simulink subsystem "PvtSubSys_HMI"  (R2020b)
settings: Solver=VariableStepAuto  StartTime=0.0  StopTime=10.0  RelTol=1e-3
undefined symbols (not defined in the file): P_HMI_LDW_LKAWarnTime, P_HMI_ObjectTypeFilter, P_HMI_WarnFormLDWReq
libraries: simulink x212, TrueDurationTime x6
(part 3 of 8)

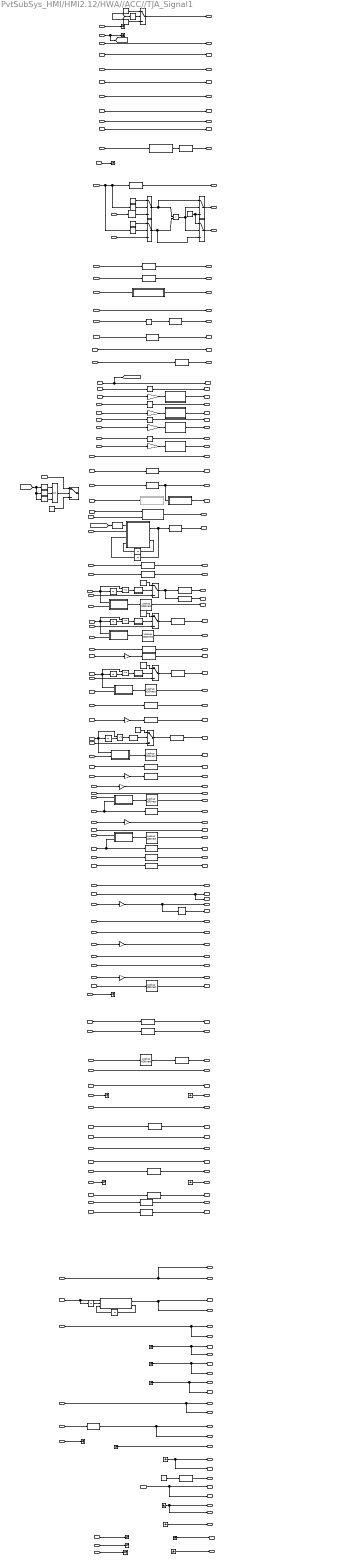
== system PvtSubSys_HMI/HMI2.12/HWA//ACC//TJA_Signal1 ==
  note: P O3目标是否存在
  note: 0x0:OFF
      | 0x1:ON
  note: 0x0:No Request
      | 0x1:Request
  note: 0x0:No Request
      | 0x1:Request
  note: 是否存在ACC 主目标PO0
  note: P O0目标是否存在
      | 仪表用ACC_RlvTgtDetn信号作为判断 目标是否存在
  note: 0=Obj_Type_INVALIDE |
      | 1=Obj_Type_UnknownType |
      | 2=Obj_Type_CAR |
      | 3=Obj_Type_TRUCK |
      | 4=Obj_Type_MOTORBIKE |
      | 5=Obj_Type_BICYCLE |
      | 6=Obj_Type_PEDESTRIAN |
      | 7=Obj_Type_GENERAL_OBJECT |
      | 8=Obj_Type_ANIMAL|
  note: DEFAULT(7)
  note: 0x0:No TakeOver request
      | 0x1:Valid TakeOver request
  note: 0x0:Fuction Not  Available
      | 0x1:Fuction Available
      | 0x2:Performance degradation(融合)
      | 0x3:Reserved
  note: 0x0:No display
      | 0x1:Distance_1 one bar
      | 0x2:Distance_2 two bars
      | 0x3:Distance_3 three bars
      | 0x4:Distance_4 four bars
      | 0x5-0x7:Resvered
  note: 0x0:No Display
      | 0x1:Override
      | 0x2:Deceleration
      | 0x3:Reserved
  note: 0x00:No display
      | 0x01:Unable to activate ACC due to speed not achive
      | 0x02:ACC active control is cancelled
      | 0x03:Resvered
      | 0x04:ACC and PEBS temporary unavailable
      | 0x05:Unable to activate ACC due to other limitation(except speed not achive)
      | 0x06:ACC and PEBS error
      | 0x07:ACC temporary unavailable
      | 0x08:Resvered
      | 0x09:Blindness
      | 0x0A-0x1F:Resvered
  note: 0x0:No display
      | 0x1:Unable to activate TJA/ICA due to other limitation
      | 0x2:TJA/ICA active control is cancelled
      | 0x3:TJA/ICA   temporarily unavailable
      | 0x4:Current IGN Cycle Function Inhibit
      | 0x5-0x7:Resvered
  note: 0x0:OFF mode
      | 0x1:Idle mode
      | 0x2:Ready mode
      | 0x3:Active
      | 0x4:Reserved
      | 0x5:Warning Level 1
      | 0x6:Warning Level 2
      | 0x7:Warning Level 3
      | 0x8:Reserved
      | 0x9:Failure
      | 0xA-0xF:Reserved
  note: 0x0:No display
      | 0x1:Unable to activate CruiseChauffer due to other limitation
      | 0x2:CruiseChauffer active control is cancelled
      | 0x3:CruiseChauffer temporarily unavailable
      | 0x4:Take over request
      | 0x5:Current IGN Cycle Function Inhibit
      | 0x6: Please Keep Attention
      | 0x7:To cross the tunnel, please take over  in time
      | 0x8:Have a branch road ahead. Please take over in time
      | 0x9-0xF:Reserved
  note: 0x0:No display
      | 0x1:TimeGap_1 1s
      | 0x2:TimeGap_2 1.4s
      | 0x3:TimeGap_3 1.8s
      | 0x4:TimeGap_4 2.1s
      | 0x5-0x7:Reserved
  note: 0x0:No object
      | 0x1:Target object detected
  note: 0x0:Not dectected
      | 0x1:Dectected
      | 0x2:Reserved
      | 0x3:Invalid
  note: 0x0:OFF mode
      | 0x1:Passive mode
      | 0x2:Active mode
      | 0x3:Reserved
      | 0x4: Failure
      | 0x5-0x7: Reserved
  note: 3 off
      | 0 off_selected
      | 1 acc_selected
      | 2 tja_seclected
      | 4 acc_on
      | 5 tja_on
  note: 0x0:No Warning
      | 0x1:Warning Level 1
      | 0x2:Warning Level 2
      | 0x3:Warning Level 3
  note: 0x0:No display
      | 0x1:Unable to activate HWA due to other limitation
      | 0x2:HWA active control is cancelled
      | 0x3:Turn off the turn light
      | 0x4:Active confirm
      | 0x5:Overtime for lane change
      | 0x6:lane change is cancelled
      | 0x7:HWA temporary unavailable
      | 0x8:Speed is too low to support lane change
      | 0x9:HWA need to restart the engine
      | 0xA:Take over request
      | 0xB: Please Keep Attention
      | 0xC:To cross the tunnel, please take over  in time
      | 0xD:Have a branch road ahead. Please take over in time
      | 0xE-0xF:Reserve
  note: FD2
      | 0x0:No display
      | 0x1:left satisfied
      | 0x2:right satisfied
      | 0x3:left not satisfied
      | 0x4:right not satisfied
      | 0x5~0x7:reserved
  note: FD2
      | 0x0:No display
      | 0x1:left
      | 0x2:right
      | 0x3:reserved
  note: 0x0:OFF mode
      | 0x1:Passive mode(Reject)
      | 0x2:Passive mode(Stand-by)
      | 0x3:Active-Control mode
      | 0x4:Brake-only mode
      | 0x5:Override
      | 0X6:Standstill
      | 0x7:Failure mode Longctrl
      | 0x8:Reserved
      | 0x9:Shut off
      | 0xA~0xF:Reserved
  note: 0x0:No Request
      | 0x1:Request
  note: ACC起步请求标志位
  note: 0x0:No request
      | 0x1:Request park Shift
      | 0x2:Invalid
      | 0x3:Reserved
  note: 1：park
      | 0：no
  note: 0x0:Not active
      | 0x1:AEB active
      | 0x2:Safestop active
      | 0x3:Reserved
  note: 0x0: No Display
      | 0x1: HOD Level 1
      | 0x2: HOD Level 2
      | 0x3: DAM Warning
      | 0x4-0x7:Resvered
  note: Diver Hands-on detection warning and
      | Driver Attention warning
  note: 0x0:Normal
      | 0x1:High sensitivity
      | 0x2:Low sensitivity
      | 0x3:Reserved
  note: 需要修改coding
  note: 状态机
  note: 0：preceding
      | 1： oncoming
  note: 前方300m（暂定）弯道曲率
  note: 0x0 00-0x1FE:Valid Value(Left bend)
      | 0x1 FF:Straightaway
      | 0x2 00-0x3FD:Valid Value((Reft bend))
      | 0x3 FE:Reserved
      | 0x3 FF:Unknown
  note: Current position curvature
  note: 当前位置道路曲率
  note: Object_Type
  note: ACC主目标：ACCTarget objective and Video Camera Fusion
      | 0x0:No Fusion
      | 0x1:Fusion
  note: 0x0:Not active
      | 0x1:Active
  note: coding值oncoming规划到Reseved
  note: 0x0:No display
      | 0x1:Automatic lane change function failure
      | 0x2-0x3:Reserve
  note: 黄色：ACC_FD2
      | 绿色：ACC_FD1
  note: 0x0=Frader前雷达
      | 0x1=Fcamera前摄像头
      | 0x2=LFRadar左前雷达
      | 0x3=RFRadar右前雷达
      | 0x4=RLRader左后雷达
      | 0x5=RRRader 右后
      | 0x6=FRadCamFusion前雷达和摄像头
      | 0x7=FRadCamLRadFusion前雷达摄像头左前
      | 0x8=FRadCamRRadFusion前雷达摄像头右前
      | 0x9=FRadCamRRadLRadFusion前雷达摄像头左前右前
      | 0x10=FRadLRadFusion 前雷达左前
      | 0x11=FRadRRadFusion前雷达右前
      | 0x12=FRadLRadRRadFusion前雷达右前左前
      | 0x13=LRadRRadFusion 右前左前
      | 0x14=OtherFusion
  note: 0x0:Unknown
      | 0x1:Emergency lane
      | 0x2:Single-lane road
      | 0x3:Left-most lane
      | 0x4:Right-most lane
      | 0x5:One of middle lanes on road with three or more lanes
      | 0x6:Reserved
      | 0x7:Invalid data
  note: Lateral distance of the second target in left lane
  note: 0x0:Unkown
      | 0x1:Sedan
      | 0x2:Truck
      | 0x3:Motorcycle
      | 0x4:Pedestrian
      | 0x5:Bicycle
      | 0x6:Reserved
      | 0x7:Invalid
  note: 0x0:Not dectected
      | 0x1:Dectected
      | 0x2:Reserved
      | 0x3:Invalid
  note: 0x0:No Request
      | 0x1:Request
  note: 0x0:No Response
      | 0X1:Response
  note: 核实后：雷达 故障的时候发invalid
  note: SpdLim_Long_Distance
  note: 0x0:OFF
      | 0X1:ON
  note: 0x0:UNDEFINED
      | 0x1:PRECEDING
      | 0x2:STATIONARY
      | 0x3:STOPPED
      | 0x4-0x7:Reserved
  note: 0x0:Unkown
      | 0x1:Sedan
      | 0x2:Truck
      | 0x3:Motorcycle
      | 0x4:Pedestrian
      | 0x5:Bicycle
      | 0x6:Reserved
      | 0x7:Invalid
  note: error=invalid
  note: 0x0:No display
      | 0x1:Distance_1 one bar
      | 0x2:Distance_2 two bars
      | 0x3:Distance_3 three bars
      | 0x4:Distance_4 four bars
      | 0x5-0x7:Resvered
  note: 0x0:off
      | 0x1:ACC selected
      | 0x2:TJA/ICA selected
      | 0x3:Off selected
      | 0x4:ACC on
      | 0x5:TJA/ICA on
      | 0x6-0x7:Reserved
  note: 0x0:no fusion
      | 0x1:fusion
  note: 0x0:OFF
      | 0x1:ON
  note: 0x0:off
      | 0x1:ACC selected
      | 0x2:TJA/ICA selected
      | 0x3:Off selected
      | 0x4:ACC on
      | 0x5:TJA/ICA on
      | 0x6-0x7:Reserved
  note: 0x0:inactive0x1:active
  note: 0x0:Unkown
      | 0x1:Sedan
      | 0x2:Truck
      | 0x3:Motorcycle
      | 0x4:Pedestrian
      | 0x5:Bicycle
      | 0x6:Reserved
      | 0x7:Invalid
  note: 0x0:No display
      | 0x1:Speed Limit Confirm Request
      | 0x2:Speed Limit Take Over Request
      | 0x3:Reduce speed on a curve(过弯安全降速)
  note: 0=Obj_MovType_INVALID |
      | 1=Obj_MovType_UNKNOWN |
      | 2=Obj_MovType_MOVING |
      | 3=Obj_MovType_STATIONARY |
      | 4=Obj_MovType_STOPPED|
      | 5= Obj_MovType_MOVING_SLOWLY
  note: 0x0:Unknown
      | 0x1:Hands off
      | 0x2:Not hands off
      | 0x3:Reserved
  note: 0x0:no request
      | 0x1:The front car has started
      | 0x2:The front car has started,Please pay attention to the road environmentahead
      | 0x3:The front car has started,please keep your attention
      | 0x4:The front car has started,please take over the car
      | 0x5-0x7:Reserved
  note: 0x0:Good
      | 0x1:Unbelievable
      | 0x2:Low
      | 0x3:Middle
      | 0x4:High Level 1
      | 0x5:High Level 2
  note: 0x0:No warning
      | 0x1:Level1 warning
      | 0x2:Level2 warning
      | 0x3:Level3 warning
      | 0x4:Level4 warning
      | 0x5:Level5 warning
      | 0x6-0x7:Reserved
  note: HWAWarnig优先级最高，可屏蔽其他两者；Handsoffwarn和DrvrSts谁高报谁，一样则报Handsoff；
  note: 0x0:Turn OFF
      | 0x1:Turn Left ON
      | 0x2:Turn Right ON
  ACCSts : Inport
  TJASts : Inport  Port=2
  HWASts : Inport  Port=3
  ACC_ModeDisp : Inport  Port=4
  TJA_ModeDisp : Inport  Port=5
  HWA_ModeDisp : Inport  Port=6
  ACCTextDisp : Inport  Port=7
  TJATextDisp : Inport  Port=8
  ALC_Resp : Inport  Port=9
  HWA_Resp : Inport  Port=10
  HWAWarningLevel : Inport  Port=11
  ACC_TimeGapSet : Inport  Port=12
  ACC_SpdSetValue : Inport  Port=13
  TJA_ACC_SelSts : Inport  Port=14
  ACC_TakeOverReq : Inport  Port=15
  ACC_HazActv : Inport  Port=16
  IntelligentCurveActive : Inport  Port=17
  fu_typeP0 : Inport  Port=18
  P0HeadingAngle : Inport  Port=19
  fu_typeP2 : Inport  Port=20
  P2HeadingAngle : Inport  Port=21
  fu_typeP3 : Inport  Port=22
  P3HeadingAngle : Inport  Port=23
  fu_typeP1 : Inport  Port=24
  P1HeadingAngle : Inport  Port=25
  DriverInloop_Monitor : Inport  Port=26
  HWA_SnvtySet_Resp : Inport  Port=27
  HWA_LaneChangeReq : Inport  Port=28
  ACC_Decel_Req : Inport  Port=29
  ACC_ISLResp : Inport  Port=30
  ICA_HandsOffSwtResp : Inport  Port=31
  targetExistP0 : Inport  Port=32
  ObjTypeP0 : Inport  Port=33
  targetExistP1 : Inport  Port=34
  ObjTypeP1 : Inport  Port=35
  dxP1 : Inport  Port=36
  ObjDYP1 : Inport  Port=37
  targetExistP2 : Inport  Port=38
  ObjTypeP2 : Inport  Port=39
  dxP2 : Inport  Port=40
  ObjDYP2 : Inport  Port=41
  targetExistP3 : Inport  Port=42
  ObjTypeP3 : Inport  Port=43
  dxP3 : Inport  Port=44
  ObjDYP3 : Inport  Port=45
  ISL_InterSysInfoDisp : Inport  Port=46
  ACC_DrvOffReq : Inport  Port=47
  IDP2 : Inport  Port=48
  IDP1 : Inport  Port=49
  IDP3 : Inport  Port=50
  ACC_Decel_ReqValue : Inport  Port=51
  ACC_ParkShiftReq : Inport  Port=52
  HCUTrqReqActive : Inport  Port=53
  CCTextDisp : Inport  Port=54
  dyP4 : Inport  Port=55
  dxP4 : Inport  Port=56
  ObjTypeP4 : Inport  Port=57
  targetExistP4 : Inport  Port=58
  dyP5 : Inport  Port=59
  dxP5 : Inport  Port=60
  ObjTypeP5 : Inport  Port=61
  targetExistP5 : Inport  Port=62
  IDP0 : Inport  Port=63
  dxP0 : Inport  Port=64
  ObjDYP0 : Inport  Port=65
  ACCTgtObjObstcl : Inport  Port=66
  ACCTgtObjExist : Inport  Port=67
  ACCTgtObjVy : Inport  Port=68
  vxRelP0 : Inport  Port=69
  axAbsGroundP0 : Inport  Port=70
  ACCTgtObjAy : Inport  Port=71
  ObjMovingStateP0 : Inport  Port=72
  Object_Orientation : Inport  Port=73
  ACCTgtObjCntAlive : Inport  Port=74
  HandsoffDetd : Inport  Port=75
  DrivingOnHighWay : Inport  Port=76
  dRoadCurvature : Inport  Port=77
  TSR_Sign_Long_Distance : Inport  Port=78
  RoadCurvatureFar : Inport  Port=79
  RampDistance : Inport  Port=80
  NavSpdLimValue : Inport  Port=81
  RoadCurvatureFarDistance : Inport  Port=82
  NavSpdLimUnit_HUT : Inport  Port=83
  TunnelDistance : Inport  Port=84
  ADAS_Posn_CurLane : Inport  Port=85
  BridgeDistance : Inport  Port=86
  ACC_SOS_Req : Inport  Port=87
  MapDataValid : Inport  Port=88
  DrvrState : Inport  Port=89
  "Inter_AEB_TgtDecel_Req " : Inport  Port=90
  Inter_FCW_Warn : Inport  Port=91
  CruiseChauffeur_ModeDisp : Inport  Port=92
  HWATextDisp : Inport  Port=93
  HandsOffWarningLevel : Inport  Port=94
  ACC_TgtObjBarDisp1 : Inport  Port=95
  ACC_LeTgtObjBarDisp1 : Inport  Port=96
  ACC_RiTgtObjBarDisp1 : Inport  Port=97
  HWA_TurnLightReq : Inport  Port=98
  ACC_DrvrOffDisp : Inport  Port=99
  100ms1 : Subsystem
  100ms2 : Subsystem
  100ms3 : Subsystem
  100ms4 : Subsystem
  ACCSts1 : InportShadow
  ACCSts2 : InportShadow
  ACCSts4 : InportShadow
  ACC_Decel_Req1 : InportShadow  Port=29
  Compare To Constant : simulink/Logic and Bit Operations/Compare To Constant  relop=~=  const=7  OutDataTypeStr=boolean
  Compare To Constant{1..6} (6 alike) : simulink/Logic and Bit Operations/Compare To Constant  relop=~=  const=0  OutDataTypeStr=boolean
  Compare To Constant10 : simulink/Logic and Bit Operations/Compare To Constant  relop===  const=7  OutDataTypeStr=boolean
  Compare To Constant7 : simulink/Logic and Bit Operations/Compare To Constant  relop===  const=3  OutDataTypeStr=boolean
  Compare To Constant8 : simulink/Logic and Bit Operations/Compare To Constant  relop===  const=5  OutDataTypeStr=boolean
  Compare To Constant9 : simulink/Logic and Bit Operations/Compare To Constant  relop===  const=6  OutDataTypeStr=boolean
  Constant{,1..2,10} (4 alike) : Constant  Value=0  OutDataTypeStr=uint8
  Constant3 : Constant
  Constant4 : Constant  Value=0
  Constant{5..8} (4 alike) : Constant  Value=0  OutDataTypeStr=boolean
  Constant9 : Constant  OutDataTypeStr=uint8
  Data Type Conversion{,1..30,34,36} (33 alike) : DataTypeConversion
  Data Type Conversion31 : DataTypeConversion  OutDataTypeStr=uint16
  Data Type Conversion32 : DataTypeConversion  OutDataTypeStr=uint16
  Data Type Conversion33 : DataTypeConversion  OutDataTypeStr=uint16
  Data Type Conversion35 : DataTypeConversion  OutDataTypeStr=uint8
  Detect Increase23 : simulink/Logic and Bit Operations/Detect Increase  vinit=0.0  OutDataTypeStr=boolean
  Direct Lookup Table (n-D){,1..3,8..9} (6 alike) : LookupNDDirect  NumberOfTableDimensions=1  Table=[7 0 1 2 3 5 4 0 0]  TableDataTypeStr=uint8
  Direct Lookup Table (n-D)10 : LookupNDDirect  NumberOfTableDimensions=1  Table=[1 0 1 2 3 4 1 2 3 4]  TableDataTypeStr=uint8
  Direct Lookup Table (n-D)4 : LookupNDDirect  NumberOfTableDimensions=1  Table=[0 0 1 2 3 1]  TableDataTypeStr=uint8
  Direct Lookup Table (n-D)5 : LookupNDDirect  NumberOfTableDimensions=1  Table=[2 1]  TableDataTypeStr=uint8
  Enlong3s : Subsystem
  Gain{,1..3} (4 alike) : Gain  Gain=-1/57.3  OutDataTypeStr=Inherit: Same as input
  Gain{4..11} (8 alike) : Gain  Gain=-1  OutDataTypeStr=Inherit: Same as input
  Ground{,1,3..8,12,14,20} (11 alike) : Ground
  HWASts1 : InportShadow  Port=3
  IDP0copy : InportShadow  Port=63
  Logical Operator : Logic  Operator=OR  Inputs=3  AllPortsSameDT=off  OutDataTypeStr=boolean
  MATLAB Function : MATLAB Function  TreatAsAtomicUnit=on
  MATLAB Function1 : MATLAB Function  TreatAsAtomicUnit=on
  MATLAB Function2 : MATLAB Function  TreatAsAtomicUnit=on
  MATLAB Function3 : MATLAB Function  Commented=on  TreatAsAtomicUnit=on
  MATLAB Function4 : MATLAB Function  TreatAsAtomicUnit=on
  MATLAB Function5 : MATLAB Function  TreatAsAtomicUnit=on
  MATLAB Function6 : MATLAB Function  TreatAsAtomicUnit=on
  MATLAB Function7 : MATLAB Function  TreatAsAtomicUnit=on
  MATLAB Function8 : MATLAB Function  TreatAsAtomicUnit=on
  MATLAB Function9 : MATLAB Function  TreatAsAtomicUnit=on
  Relational Operator : RelationalOperator  Operator=>  OutDataTypeStr=boolean  RndMeth=Simplest
  Relational Operator{1..4} (4 alike) : RelationalOperator  Operator=~=  OutDataTypeStr=boolean  RndMeth=Simplest
  Signal Copy : SignalConversion  OverrideOpt=off
  Subsystem : Subsystem
  Subsystem1 : Subsystem
  Subsystem2 : Subsystem
  Subsystem3 : Subsystem
  Subsystem4 : Subsystem
  Subsystem5 : Subsystem
  Switch{,1..8} (9 alike) : Switch  Criteria=u2 ~= 0
  Switch9 : Switch  Criteria=u2 > Threshold
  Terminator{,1..6,16,18,22} (10 alike) : Terminator
  Unit Delay{,1..7} (8 alike) : UnitDelay  SampleTime=-1  HasFrameUpgradeWarning=on
  fu_typeP4 : InportShadow  Port=18
  vxRelP01 : InportShadow  Port=69
  ALC_InterSysInfoDisp : Outport
  ACC_ModDisp : Outport  Port=2
  TJA_ICA_ModDisp : Outport  Port=3
  HWA_InterSysInfoDisp : Outport  Port=4
  HWA_ModDisp : Outport  Port=5
  ACC_InterSysInfoDisp : Outport  Port=6
  TJA_ICA_InterSysInfoDisp : Outport  Port=7
  ALCResp : Outport  Port=8
  HWAResp : Outport  Port=9
  HWAwarning : Outport  Port=10
  ACCTimeGapSet : Outport  Port=11
  ACCSpdSetValue : Outport  Port=12
  TJA_ACCSelSts : Outport  Port=13
  ACCTakeOverReq : Outport  Port=14
  ACC_FctSts : Outport  Port=15
  ACCTgtObjBarDisp : Outport  Port=16
  Longctrl_HazActv : Outport  Port=17
  IntelligentCurveAct : Outport  Port=18
  ACC_RlvTgtfusion : Outport  Port=19
  ACC_RlvTgtHeading : Outport  Port=20
  ACC_LeTgtfusion : Outport  Port=21
  ACC_LeTgtHeading : Outport  Port=22
  ACC_RiTgtfusion : Outport  Port=23
  ACC_RiTgtHeading : Outport  Port=24
  ACC_PotentialTgtfusion : Outport  Port=25
  ACC_PotentialTgtHeading : Outport  Port=26
  ADAS_DriverInloop_Monitor : Outport  Port=27
  HWASnvtySetResp : Outport  Port=28
  HWA_Lane_ChangeReq : Outport  Port=29
  HWA_LaneChange : Outport  Port=30
  ACC_EgoStatus : Outport  Port=31
  ISL_Resp : Outport  Port=32
  ICA_HandsOffResp : Outport  Port=33
  ACC_ObjDetecte : Outport  Port=34
  ACC_RlvTgtDetn : Outport  Port=35
  ACC_RlvTgtTyp : Outport  Port=36
  ACC_PotentialTgtDetn : Outport  Port=37
  ACC_PotentialTgtTyp : Outport  Port=38
  ACC_PotentialTgtDx : Outport  Port=39
  ACC_PotentialTgtDy : Outport  Port=40
  ACC_LeTargrtDection : Outport  Port=41
  ACC_LeTgtTyp : Outport  Port=42
  ACC_LeTgtDx : Outport  Port=43
  ACC_LeTgtDy : Outport  Port=44
  ACC_RiTargrtDetn : Outport  Port=45
  ACC_RiTgtTyp : Outport  Port=46
  ACC_RiTgtDx : Outport  Port=47
  ACC_RiTgtDy : Outport  Port=48
  ISLInterSysInfoDisp : Outport  Port=49
  ACCLeTgtObjBarDisp : Outport  Port=50
  ACCRiTgtObjBarDisp : Outport  Port=51
  Longctrl_DrvOFF_Req_DVR : Outport  Port=52
  Request_driveoff : Outport  Port=53
  Longctrl_ModSts_DVR : Outport  Port=54
  Longctrl_Decel_Req_DVR : Outport  Port=55
  Longctrl_EngTrqReq_DVR : Outport  Port=56
  Longctrl_EngTrqReqActive_DVR : Outport  Port=57
  Longctrl_DecelToStopReq_DVR : Outport  Port=58
  Longctrl_Decel_ReqValue_DVR : Outport  Port=59
  Longctrl_ParkShiftReq_DVR : Outport  Port=60
  Longctrl_VehHldReq_DVR : Outport  Port=61
  Longctrl_HCUTrqReqActive_DVR : Outport  Port=62
  Longctrl_HCUTrqReq_DVR : Outport  Port=63
  ACC_LeTgt_02_Dy : Outport  Port=64
  ACC_LeTgt_02_Dx : Outport  Port=65
  ACC_LeTgt_02_Typ : Outport  Port=66
  ACC_LeTargrt_02_Detn : Outport  Port=67
  ACC_RiTgt_02_Dy : Outport  Port=68
  ACC_RiTgt_02_Dx : Outport  Port=69
  ACC_RiTgt_02_Typ : Outport  Port=70
  ACC_RiTargrt_02_Detn : Outport  Port=71
  ACC_RlvTgtDx : Outport  Port=72
  ACC_RlvTgtDy : Outport  Port=73
  Longctrl_DrvOFF_Req : Outport  Port=74
  Longctrl_ModSts : Outport  Port=75
  Longctrl_Decel_Req : Outport  Port=76
  Longctrl_EngTrqReq : Outport  Port=77
  Longctrl_EngTrqReqActive : Outport  Port=78
  Longctrl_DecelToStopReq : Outport  Port=79
  Longctrl_Decel_ReqValue : Outport  Port=80
  Longctrl_ParkShiftReq : Outport  Port=81
  ActualTargetSpeed : Outport  Port=82
  Longctrl_VehHldReq : Outport  Port=83
  ACC_CRInterface : Outport  Port=84
  Longctrl_HCUTrqReqActive : Outport  Port=85
  Longctrl_HCUTrqReq : Outport  Port=86
  Longctrl_FuelCutOffPrevn : Outport  Port=87
  ACCTgtObjID : Outport  Port=88
  ACCTgtObjDx : Outport  Port=89
  ACCTgtObjDy : Outport  Port=90
  ACC_TgtObjObstcl : Outport  Port=91
  ACC_TgtObjExist : Outport  Port=92
  ACC_TgtObjVy : Outport  Port=93
  ACCTgtObjVx : Outport  Port=94
  ACCTgtObjAx : Outport  Port=95
  ACC_TgtObjAy : Outport  Port=96
  ACCTgtObjState : Outport  Port=97
  ACCTgtObjVideoCfmd : Outport  Port=98
  ACC_TgtObjCntAlive : Outport  Port=99
  Handsoff_Detd : Outport  Port=100
  DrvgOnHiWay : Outport  Port=101
  RoadCrvt : Outport  Port=102
  SpdLimitDst : Outport  Port=103
  RoadCrvtFar : Outport  Port=104
  RampDst : Outport  Port=105
  SpdLimit : Outport  Port=106
  CurveDst : Outport  Port=107
  NavSpdLimUnit : Outport  Port=108
  TunnelDst : Outport  Port=109
  Drvg_OnRiLane : Outport  Port=110
  BrdgDst : Outport  Port=111
  ACC_SOSReq : Outport  Port=112
  Map_DataValid : Outport  Port=113
  DrvrSts : Outport  Port=114
  CruCha_ModDisp : Outport  Port=115
  CruChar_InterSysInfoDisp : Outport  Port=116
  IFC_Handsoffwarn : Outport  Port=117
  HWA_TurnLightReqout : Outport  Port=118
  wires:
  Unit Delay7/1 -> MATLAB Function9/4(countk1)
  MATLAB Function9/2(count) -> Unit Delay7/1
  Unit Delay6/1 -> MATLAB Function9/3(yk1)
  Detect Increase23/1 -> MATLAB Function9/1(IntelligentCurveActive)
  ISL_InterSysInfoDisp/1 -> MATLAB Function9/2(ISL_InterSysInfoDisp)
  [IntelligentCurveActive] -> Detect Increase23/1
  MATLAB Function9/1(y) -> Data Type Conversion24/1, Unit Delay6/1
  Constant10/1 -> Switch9/3
  Constant9/1 -> Switch9/1
  Compare To Constant10/1 -> Switch9/2
  [HWASts] -> Compare To Constant10/1
  Unit Delay5/1 -> MATLAB Function/2(ACCStsK1)
  Unit Delay4/1 -> MATLAB Function/3(CntK1)
  MATLAB Function/2(Cnt) -> Unit Delay4/1
  Enlong3s/1(Out1) -> Data Type Conversion27/1
  HWA_LaneChangeReq/1 -> Data Type Conversion12/1
  Constant4/1 -> Switch4/3
  Logical Operator/1 -> Switch4/2
  Compare To Constant9/1 -> Logical Operator/3
  Compare To Constant8/1 -> Logical Operator/2
  Compare To Constant7/1 -> Logical Operator/1
  [HWASts] -> Compare To Constant7/1, Compare To Constant8/1, Compare To Constant9/1
  Data Type Conversion36/1 -> ACC_CRInterface/1
  MATLAB Function7/1(Angle) -> ACC_PotentialTgtHeading/1
  MATLAB Function6/1(Angle) -> ACC_RiTgtHeading/1
  MATLAB Function5/1(Angle) -> ACC_LeTgtHeading/1
  MATLAB Function4/1(Angle) -> ACC_RlvTgtHeading/1
  Gain3/1 -> MATLAB Function7/1(AngRaw)
  Gain2/1 -> MATLAB Function6/1(AngRaw)
  Gain1/1 -> MATLAB Function5/1(AngRaw)
  Gain/1 -> MATLAB Function4/1(AngRaw)
  Subsystem5/1(Out1) -> Direct Lookup Table (n-D)9/1
  Subsystem4/1(Out1) -> Direct Lookup Table (n-D)8/1
  Subsystem3/1(Out1) -> Direct Lookup Table (n-D)3/1
  Subsystem2/1(Out1) -> Direct Lookup Table (n-D)2/1
  Subsystem1/1(Out1) -> Direct Lookup Table (n-D)1/1
  Subsystem/1(Out1) -> Direct Lookup Table (n-D)/1
  Signal Copy/1 -> ACCTgtObjDy/1
  Compare To Constant6/1 -> ACC_PotentialTgtfusion/1
  Direct Lookup Table (n-D)10/1 -> Switch1/3
  targetExistP0/1 -> Switch8/3
  IDP0copy/1 -> Unit Delay3/1, Relational Operator4/1, Subsystem/1(id)
  Unit Delay3/1 -> Relational Operator4/2
  Relational Operator4/1 -> 100ms4/1(In1)
  Constant8/1 -> Switch8/1
  100ms4/1(Out1) -> Switch8/2
  Switch7/1 -> Data Type Conversion15/1
  100ms3/1(Out1) -> Switch7/2
  Constant7/1 -> Switch7/1
  Relational Operator3/1 -> 100ms3/1(In1)
  Unit Delay2/1 -> Relational Operator3/2
  IDP1/1 -> Relational Operator3/1, Unit Delay2/1, Subsystem1/1(id)
  targetExistP1/1 -> Switch7/3
  Switch6/1 -> Data Type Conversion18/1
  targetExistP2/1 -> Switch6/3
  IDP2/1 -> Relational Operator2/1, Unit Delay1/1, Subsystem2/1(id)
  Unit Delay1/1 -> Relational Operator2/2
  Relational Operator2/1 -> 100ms2/1(In1)
  Constant6/1 -> Switch6/1
  100ms2/1(Out1) -> Switch6/2
  Switch5/1 -> Data Type Conversion21/1
  100ms1/1(Out1) -> Switch5/2
  Constant5/1 -> Switch5/1
  Relational Operator1/1 -> 100ms1/1(In1)
  Unit Delay/1 -> Relational Operator1/2
  IDP3/1 -> Relational Operator1/1, Unit Delay/1, Subsystem3/1(id)
  Gain11/1 -> ACC_TgtObjAy/1
  Gain10/1 -> ACC_TgtObjVy/1
  Gain9/1 -> Signal Copy/1, ACC_RlvTgtDy/1
  Gain8/1 -> ACC_RiTgt_02_Dy/1
  Gain7/1 -> ACC_LeTgt_02_Dy/1
  Gain6/1 -> Data Type Conversion23/1
  Gain5/1 -> Data Type Conversion20/1
  Gain4/1 -> Data Type Conversion17/1
  P1HeadingAngle/1 -> Gain3/1
  P3HeadingAngle/1 -> Gain2/1
  P2HeadingAngle/1 -> Gain1/1
  Data Type Conversion35/1 -> HWA_TurnLightReqout/1
  HWA_TurnLightReq/1 -> Data Type Conversion35/1
  ACCSts/1 -> Terminator6/1
  ACC_DrvrOffDisp/1 -> Enlong3s/1(In1)
  Data Type Conversion34/1 -> ACCTgtObjBarDisp/1
  Data Type Conversion33/1 -> BrdgDst/1
  Data Type Conversion32/1 -> TunnelDst/1
  Data Type Conversion31/1 -> RampDst/1
  Switch2/1 -> IFC_Handsoffwarn/1
  Constant2/1 -> Switch3/3, Switch2/1
  Relational Operator/1 -> Switch2/2, Switch3/2
  Switch/1 -> Switch2/3, Relational Operator/2
  Switch1/1 -> Switch3/1, Relational Operator/1
  Switch3/1 -> DrvrSts/1
  Compare To Constant2/1 -> Switch/2
  Compare To Constant1/1 -> Switch1/2
  Constant1/1 -> Switch1/1
  Constant/1 -> Switch/1
  HWAWarningLevel/1 -> Compare To Constant1/1, Data Type Conversion7/1, Compare To Constant2/1
  HandsOffWarningLevel/1 -> Switch/3
  Constant3/1 -> Data Type Conversion36/1
  Direct Lookup Table (n-D)5/1 -> Data Type Conversion3/1
  Direct Lookup Table (n-D)4/1 -> ACCTgtObjState/1
  Direct Lookup Table (n-D)3/1 -> ACC_RiTgtTyp/1
  Direct Lookup Table (n-D)2/1 -> ACC_LeTgtTyp/1
  Direct Lookup Table (n-D)1/1 -> ACC_PotentialTgtTyp/1
  HWASts/1 -> Terminator2/1, [HWASts]
  TJATextDisp/1 -> TJA_ICA_InterSysInfoDisp/1
  ACCTextDisp/1 -> ACC_InterSysInfoDisp/1
  HWATextDisp/1 -> HWA_InterSysInfoDisp/1
  Data Type Conversion28/1 -> ACC_RlvTgtDetn/1
  Data Type Conversion14/1 -> ACC_ObjDetecte/1
  Data Type Conversion27/1 -> Request_driveoff/1
  ACC_DrvOffReq/1 -> Longctrl_DrvOFF_Req/1, Longctrl_DrvOFF_Req_DVR/1
  Data Type Conversion26/1 -> ACCRiTgtObjBarDisp/1
  Data Type Conversion25/1 -> ACCLeTgtObjBarDisp/1
  Data Type Conversion24/1 -> ISLInterSysInfoDisp/1
  Data Type Conversion23/1 -> ACC_RiTgtDy/1
  Data Type Conversion22/1 -> ACC_RiTgtDx/1
  Data Type Conversion21/1 -> ACC_RiTargrtDetn/1
  Data Type Conversion20/1 -> ACC_LeTgtDy/1
  Data Type Conversion19/1 -> ACC_LeTgtDx/1
  Data Type Conversion18/1 -> ACC_LeTargrtDection/1
  Data Type Conversion17/1 -> ACC_PotentialTgtDy/1
  Data Type Conversion16/1 -> ACC_PotentialTgtDx/1
  Data Type Conversion15/1 -> ACC_PotentialTgtDetn/1
  Switch8/1 -> Data Type Conversion14/1, Data Type Conversion28/1
  Data Type Conversion13/1 -> HWASnvtySetResp/1
  Data Type Conversion12/1 -> HWA_Lane_ChangeReq/1, MATLAB Function8/1(Lane_ChangeReq)
  Data Type Conversion11/1 -> ACC_FctSts/1
  Data Type Conversion10/1 -> ICA_HandsOffResp/1
  Data Type Conversion9/1 -> ISL_Resp/1
  Data Type Conversion8/1 -> ACCTimeGapSet/1
  Data Type Conversion7/1 -> HWAwarning/1
  Data Type Conversion6/1 -> ACCSpdSetValue/1
  IntelligentCurveActive/1 -> IntelligentCurveAct/1, [IntelligentCurveActive]
  Data Type Conversion5/1 -> Map_DataValid/1
  Data Type Conversion4/1 -> ACC_SOSReq/1
  Data Type Conversion3/1 -> Handsoff_Detd/1
  Data Type Conversion2/1 -> ACC_TgtObjCntAlive/1
  Data Type Conversion1/1 -> ACCTgtObjVideoCfmd/1
  Data Type Conversion/1 -> Longctrl_ParkShiftReq/1, Longctrl_ParkShiftReq_DVR/1
  Data Type Conversion30/1 -> ACC_RiTargrt_02_Detn/1
  targetExistP5/1 -> Data Type Conversion30/1, Subsystem5/2(targetExist)
  ObjTypeP5/1 -> Subsystem5/1(ObjType)
  Direct Lookup Table (n-D)9/1 -> ACC_RiTgt_02_Typ/1
  Data Type Conversion29/1 -> ACC_LeTargrt_02_Detn/1
  Direct Lookup Table (n-D)8/1 -> ACC_LeTgt_02_Typ/1
  targetExistP4/1 -> Data Type Conversion29/1, Subsystem4/2(targetExist)
  ObjTypeP4/1 -> Subsystem4/1(ObjType)
  dxP5/1 -> ACC_RiTgt_02_Dx/1
  dyP5/1 -> Gain8/1
  dxP4/1 -> ACC_LeTgt_02_Dx/1
  dyP4/1 -> Gain7/1
  Switch9/1 -> ALC_InterSysInfoDisp/1
  fu_typeP1/1 -> Compare To Constant6/1
  Compare To Constant5/1 -> ACC_RiTgtfusion/1
  Compare To Constant4/1 -> ACC_LeTgtfusion/1
  Compare To Constant3/1 -> ACC_RlvTgtfusion/1
  fu_typeP3/1 -> Compare To Constant5/1
  fu_typeP2/1 -> Compare To Constant4/1
  fu_typeP0/1 -> Compare To Constant3/1
  P0HeadingAngle/1 -> Gain/1
  Ground20/1 -> Longctrl_VehHldReq/1, Longctrl_VehHldReq_DVR/1
  HCUTrqReqActive/1 -> Longctrl_HCUTrqReqActive_DVR/1, Longctrl_HCUTrqReqActive/1
  Ground3/1 -> Longctrl_HCUTrqReq/1, Longctrl_HCUTrqReq_DVR/1
  Ground12/1 -> Longctrl_FuelCutOffPrevn/1
  TJASts/1 -> Terminator22/1
  ALC_Resp/1 -> ALCResp/1
  ACC_RiTgtObjBarDisp1/1 -> Data Type Conversion26/1
  ACC_LeTgtObjBarDisp1/1 -> Data Type Conversion25/1
  HWASts1/1 -> MATLAB Function3/1(HWASts)
  vxRelP01/1 -> Terminator18/1
  CruiseChauffeur_ModeDisp/1 -> Terminator16/1
  MATLAB Function/1(Longctrl_ModSts) -> Longctrl_ModSts_DVR/1, Longctrl_ModSts/1
  Ground14/1 -> ActualTargetSpeed/1
  DriverInloop_Monitor/1 -> ADAS_DriverInloop_Monitor/1
  HWA_SnvtySet_Resp/1 -> Data Type Conversion13/1
  CCTextDisp/1 -> Switch4/1
  MATLAB Function1/1(EgoStatus) -> ACC_EgoStatus/1
  ACC_Decel_Req/1 -> MATLAB Function1/2(DecelReq)
  ACCSts2/1 -> MATLAB Function1/1(ACCSts)
  ICA_HandsOffSwtResp/1 -> Data Type Conversion10/1
  ACC_ISLResp/1 -> Data Type Conversion9/1
  Object_Orientation/1 -> Terminator5/1
  Ground5/1 -> SpdLimitDst/1
  TSR_Sign_Long_Distance/1 -> Terminator4/1
  ADAS_Posn_CurLane/1 -> Terminator3/1
  Ground4/1 -> Drvg_OnRiLane/1
  Inter_FCW_Warn/1 -> Terminator1/1
  "Inter_AEB_TgtDecel_Req "/1 -> Terminator/1
  Ground1/1 -> CruChar_InterSysInfoDisp/1
  Ground/1 -> CruCha_ModDisp/1
  DrvrState/1 -> Direct Lookup Table (n-D)10/1
  MapDataValid/1 -> Data Type Conversion5/1
  ACC_SOS_Req/1 -> Data Type Conversion4/1
  BridgeDistance/1 -> Data Type Conversion33/1
  TunnelDistance/1 -> Data Type Conversion32/1
  NavSpdLimUnit_HUT/1 -> NavSpdLimUnit/1
  RoadCurvatureFarDistance/1 -> CurveDst/1
  NavSpdLimValue/1 -> SpdLimit/1
  RampDistance/1 -> Data Type Conversion31/1
  RoadCurvatureFar/1 -> RoadCrvtFar/1
  dRoadCurvature/1 -> RoadCrvt/1
  DrivingOnHighWay/1 -> DrvgOnHiWay/1
  HandsoffDetd/1 -> Direct Lookup Table (n-D)5/1
  ACCTgtObjCntAlive/1 -> Data Type Conversion2/1
  fu_typeP4/1 -> Data Type Conversion1/1
  ObjMovingStateP0/1 -> Direct Lookup Table (n-D)4/1
  ACCTgtObjAy/1 -> Gain11/1
  axAbsGroundP0/1 -> ACCTgtObjAx/1
  vxRelP0/1 -> ACCTgtObjVx/1
  ACCTgtObjVy/1 -> Gain10/1
  ACCTgtObjExist/1 -> ACC_TgtObjExist/1
  ACCTgtObjObstcl/1 -> ACC_TgtObjObstcl/1
  IDP0/1 -> ACCTgtObjID/1
  HWA_Resp/1 -> HWAResp/1
  ACC_HazActv/1 -> Longctrl_HazActv/1
  ACC_ParkShiftReq/1 -> Data Type Conversion/1
  ACC_Decel_ReqValue/1 -> Longctrl_Decel_ReqValue/1, Longctrl_Decel_ReqValue_DVR/1
  Ground8/1 -> Longctrl_DecelToStopReq/1, Longctrl_DecelToStopReq_DVR/1
  Ground6/1 -> Longctrl_EngTrqReqActive/1, Longctrl_EngTrqReqActive_DVR/1
  Ground7/1 -> Longctrl_EngTrqReq/1, Longctrl_EngTrqReq_DVR/1
  ACC_Decel_Req1/1 -> Longctrl_Decel_Req/1, Longctrl_Decel_Req_DVR/1
  ACCSts4/1 -> MATLAB Function/1(ACCSts), Unit Delay5/1
  ObjTypeP3/1 -> Subsystem3/2(ObjType)
  targetExistP3/1 -> Switch5/3
  ObjTypeP2/1 -> Subsystem2/2(ObjType)
  ObjTypeP1/1 -> Subsystem1/2(ObjType)
  Direct Lookup Table (n-D)/1 -> ACC_RlvTgtTyp/1
  ObjTypeP0/1 -> Subsystem/2(ObjType)
  MATLAB Function8/1(LaneChange) -> HWA_LaneChange/1
  ACC_TimeGapSet/1 -> Data Type Conversion8/1
  ObjDYP3/1 -> Gain6/1
  dxP3/1 -> Data Type Conversion22/1
  ObjDYP2/1 -> Gain5/1
  dxP2/1 -> Data Type Conversion19/1
  ObjDYP1/1 -> Gain4/1
  dxP1/1 -> Data Type Conversion16/1
  ObjDYP0/1 -> Gain9/1
  dxP0/1 -> ACC_RlvTgtDx/1, ACCTgtObjDx/1  "m"
  HWA_ModeDisp/1 -> HWA_ModDisp/1
  TJA_ModeDisp/1 -> TJA_ICA_ModDisp/1
  ACC_TgtObjBarDisp1/1 -> Data Type Conversion34/1
  Compare To Constant/1 -> Data Type Conversion11/1
  ACCSts1/1 -> Compare To Constant/1
  ACC_TakeOverReq/1 -> ACCTakeOverReq/1
  MATLAB Function2/1(y) -> TJA_ACCSelSts/1
  TJA_ACC_SelSts/1 -> MATLAB Function2/1(TJA_ACC_SelSts)
  ACC_SpdSetValue/1 -> Data Type Conversion6/1
  ACC_ModeDisp/1 -> ACC_ModDisp/1
